simulink model "con_lac_don_r2015a"  (R2016b)
settings: Solver=ode4  StartTime=0.0  StopTime=10.0  FixedStep=0.001  RelTol=1e-3
settings Model: Creator=ryell  LastModifiedBy=ADMIN
settings OptimizationCC: LifeSpan=inf
settings DebuggingCC: SFExecutionAtInitializationDiag=none
settings HardwareCC: ProdBitPerSizeT=32  ProdBitPerPtrDiffT=32  ProdWordSize=32  ProdHWDeviceType=Specified

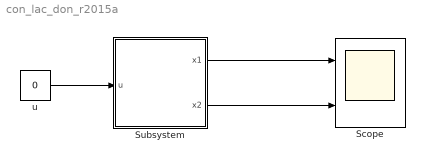
== system con_lac_don_r2015a ==
  Scope : Scope  NumInputPorts=2
  Subsystem : Subsystem  mask{g=9.81, l=0.2, m=0.5, B=0.05, x1_init=pi, x2_init=0.01}
      mask prompts: g "Gia toc trong truong"; l "Chieu dai thanh treo"; m "Khoi luong vat nang"; B "He so ma sat"; x1_init "Gia tri goc ban dau"; x2_init "Gia tri van toc goc ban dau"
  u : Constant  Value=0
  wires:
  u/1 -> Subsystem/1(u)
  Subsystem/1(x1) -> Scope/1
  Subsystem/2(x2) -> Scope/2

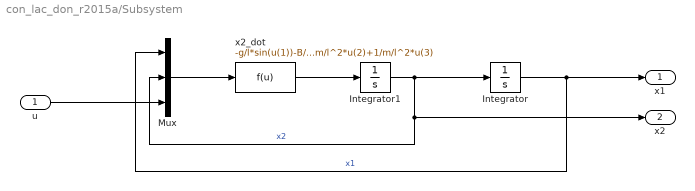
== system con_lac_don_r2015a/Subsystem ==
  u : Inport
  Integrator : Integrator  InitialCondition=x1_init
  Integrator1 : Integrator  InitialCondition=x2_init
  Mux : Mux  Inputs=3
  x2_dot : Fcn  Expr=-g/l*sin(u(1))-B/m/l^2*u(2)+1/m/l^2*u(3)
  x1 : Outport
  x2 : Outport  Port=2
  wires:
  Integrator1/1 -> x2/1, Mux/2, Integrator/1  "x2"
  u/1 -> Mux/3
  x2_dot/1 -> Integrator1/1
  Integrator/1 -> x1/1, Mux/1  "x1"
  Mux/1 -> x2_dot/1
